simulink model "tutorial26_kinematics"  (R2025a)
settings: Solver=VariableStepAuto  StartTime=0.0  StopTime=10.0  RelTol=1e-3
settings Model: Creator=xing2  LastModifiedBy=xing2

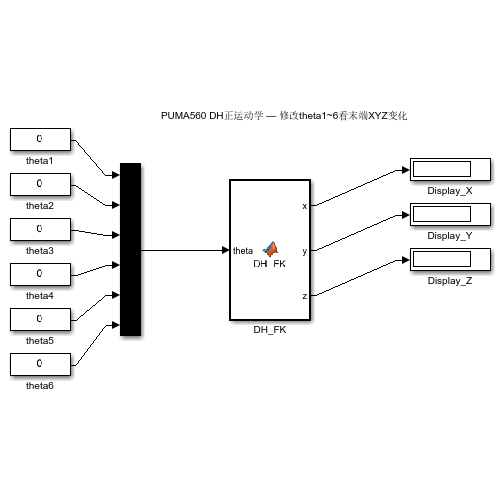
[thumbnail: Simulink's stored preview of the top-level diagram]
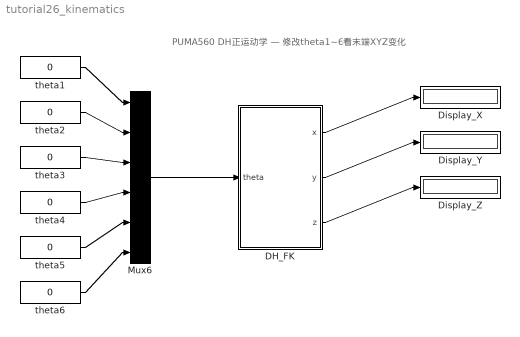
== system tutorial26_kinematics ==
  note: PUMA560 DH正运动学 — 修改theta1~6看末端XYZ变化
  DH_FK : MATLAB Function  TreatAsAtomicUnit=on
  Display_X : Display
  Display_Y : Display
  Display_Z : Display
  Mux6 : Mux  Inputs=6
  theta{1..6} (6 alike) : Constant  Value=0
  wires:
  theta1/1 -> Mux6/1
  theta2/1 -> Mux6/2
  theta3/1 -> Mux6/3
  theta4/1 -> Mux6/4
  theta5/1 -> Mux6/5
  theta6/1 -> Mux6/6
  Mux6/1 -> DH_FK/1(theta)
  DH_FK/1(x) -> Display_X/1
  DH_FK/2(y) -> Display_Y/1
  DH_FK/3(z) -> Display_Z/1

== matlab function tutorial26_kinematics/DH_FK ==
  data: x output; theta input; y output; z output
function [x,y,z] = DH_FK(theta)
% PUMA560 正运动学：关节角 → 末端XYZ
a     = [0; 0.4318; 0.0203; 0; 0; 0];
alpha = [pi/2; 0; -pi/2; pi/2; -pi/2; 0];
d     = [0.67183; 0; 0.15005; 0.4318; 0; 0.2];
T = eye(4);
for i = 1:6
    ct = cos(theta(i)); st = sin(theta(i));
    ca = cos(alpha(i)); sa = sin(alpha(i));
    T = T * [ct, -st*ca,  st*sa, a(i)*ct;
             st,  ct*ca, -ct*sa, a(i)*st;
              0,     sa,     ca,    d(i);
              0,      0,      0,       1];
end
x = T(1,4); y = T(2,4); z = T(3,4);
